simulink model "CoastdownCaCum1AQ_Ver2"  (R2024b)
settings: Solver=FixedStepAuto  StartTime=0  StopTime=14.2  FixedStep=0.2  RelTol=1e-3  AbsTol=1e-3  EnableMultiTasking=on
values from neighbouring files (symbols this model uses):
  a01 = 0.2657    [BCS_CoastdownCaCum1AQ_Ver2_lan2.mat]    (also in BCS_CoastdownCaCum2AQ_Ver2_lan2.mat)
  a02 = 0.0601    [BCS_CoastdownCaCum1AQ_Ver2_lan2.mat]    (also in BCS_CoastdownCaCum2AQ_Ver2_lan2.mat)
  a11 = 0.0614452785671    [BCS_CoastdownCaCum1AQ_Ver2_lan2.mat]    (also in BCS_CoastdownCaCum2AQ_Ver2_lan2.mat = 0.063131954008; CodeSosanhtonhaophatsinh_coastdown.m = alpha(1,1))
  a12 = 0.00726010495763    [BCS_CoastdownCaCum1AQ_Ver2_lan2.mat]    (also in BCS_CoastdownCaCum2AQ_Ver2_lan2.mat = 0.00749561097786; CodeSosanhtonhaophatsinh_coastdown.m = alpha(1,3))
  b01 = 6.7129    [BCS_CoastdownCaCum1AQ_Ver2_lan2.mat]    (also in BCS_CoastdownCaCum2AQ_Ver2_lan2.mat)
  b02 = 8.2494    [BCS_CoastdownCaCum1AQ_Ver2_lan2.mat]    (also in BCS_CoastdownCaCum2AQ_Ver2_lan2.mat)
  b11 = 1.46186355306    [BCS_CoastdownCaCum1AQ_Ver2_lan2.mat]    (also in BCS_CoastdownCaCum2AQ_Ver2_lan2.mat = 1.7584586215; CodeSosanhtonhaophatsinh_coastdown.m = alpha(1,2))
  b12 = 0.148893725861    [BCS_CoastdownCaCum1AQ_Ver2_lan2.mat]    (also in BCS_CoastdownCaCum2AQ_Ver2_lan2.mat = 0.267310835842; CodeSosanhtonhaophatsinh_coastdown.m = alpha(1,4))
  J_bx = 0.2412    [BCS_CoastdownCaCum1AQ_Ver2_lan2.mat]    (also in BCS_CoastdownCaCum2AQ_Ver2_lan2.mat)
  J_cl = 1.2576    [BCS_CoastdownCaCum1AQ_Ver2_lan2.mat]    (also in BCS_CoastdownCaCum2AQ_Ver2_lan2.mat)
  r_bx = 0.236102    [BCS_CoastdownCaCum1AQ_Ver2_lan2.mat]    (also in BCS_CoastdownCaCum2AQ_Ver2_lan2.mat = 0.235146)
  r_cl = 0.1    [BCS_CoastdownCaCum1AQ_Ver2_lan2.mat]    (also in BCS_CoastdownCaCum2AQ_Ver2_lan2.mat)
  Trr = 0.35615623487    [BCS_CoastdownCaCum1AQ_Ver2_lan2.mat]    (also in BCS_CoastdownCaCum2AQ_Ver2_lan2.mat = 0.370900243988; CodeSosanhtonhaophatsinh_coastdown.m = alpha(1,5))
  w_cl_initial = 55.8852681159    [BCS_CoastdownCaCum1AQ_Ver2_lan2.mat]    (also in BCS_CoastdownCaCum2AQ_Ver2_lan2.mat = 55.880555727; CodeSosanhtonhaophatsinh_coastdown.m = n_cl_tn(1,1)*2*pi()/60)
undefined symbols (not defined in the file or in its folder): rad, s
libraries: aerolibconvert2 x2, SignalEditorBlockLib x1
settings Model: Creator=Admin  LastModifiedBy=Legion
settings SolverCC: AutoScaleAbsTol=off  AlgebraicLoopSolver=TrustRegion  MaxZcPerStep=1
settings DataIOCC: LimitDataPoints=on  MaxDataPoints=10000
settings OptimizationCC: ReuseModelBlockBuffer=off  LifeSpan=inf
settings DebuggingCC: UnconnectedInputMsg=warning  UnconnectedOutputMsg=warning  UnconnectedLineMsg=warning  AllowSymbolicDim=off  SubsystemReferenceDiagnosticForUnitTest=warning  SFUnexpectedBacktrackingDiag=warning  SFNoUnconditionalDefaultTransitionDiag=warning  SFExecutionAtInitializationDiag=none  ArithmeticOperatorsInVariantConditions=warning
settings ModelReferenceCC: EnableRefExpFcnMdlSchedulingChecks=on
settings SFSimCC: SimUseLocalCustomCode=off  CustomCodeUndefinedFunction=UseInterfaceOnly
settings RTWCC: RTWUseLocalCustomCode=off  GPUComputeCapability=3.5  DLArmComputeVersion=19.05
settings CodeAppCC: StateflowObjectComments=on
settings GRTTargetCC: TargetLangStandard=C89/C90 (ANSI)
settings ConfigComp: CovMetricSettings=dw  CovSaveCumulativeToWorkspaceVar=on  CovSaveSingleToWorkspaceVar=on  CovExternalEMLEnable=off  CovSFcnEnable=off
settings SimscapeCC: SimscapeLogType=all  SimscapeLogSimulationStatistics=on  SimscapeLogDataHistory=10000

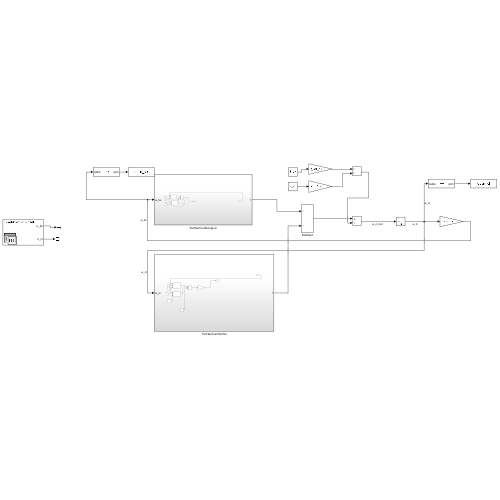
[thumbnail: Simulink's stored preview of the top-level diagram]
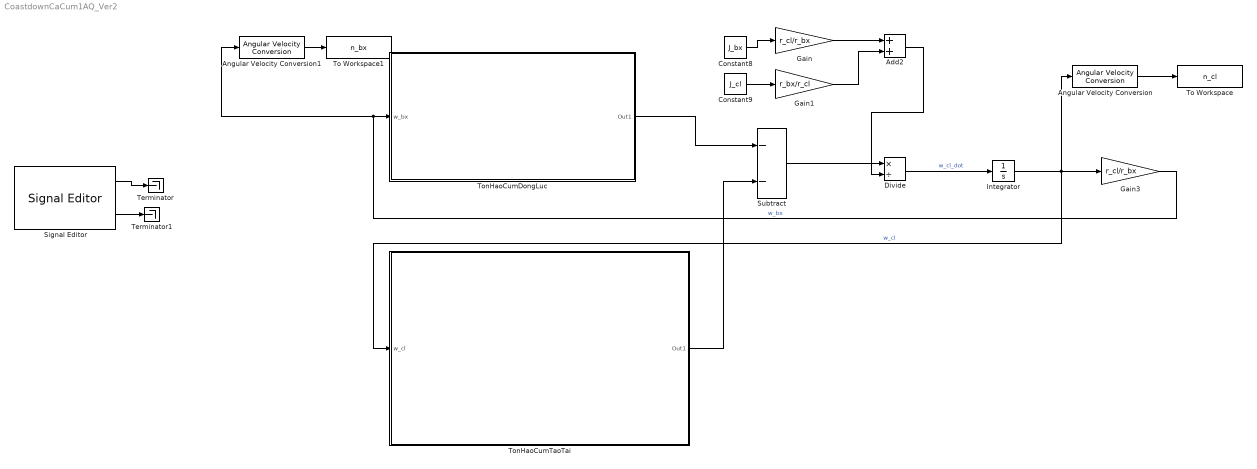
== system CoastdownCaCum1AQ_Ver2 ==
  Add2 : Sum
  Angular Velocity Conversion : aerolibconvert2/Angular Velocity Conversion  IU=rad/s  OU=rpm
  Angular Velocity Conversion1 : aerolibconvert2/Angular Velocity Conversion  IU=rad/s  OU=rpm
  Constant8 : Constant  Value=J_bx
  Constant9 : Constant  Value=J_cl  VectorParams1D=off
  Divide : Product  Inputs=*/
  Gain : Gain  Gain=r_cl/r_bx
  Gain1 : Gain  Gain=r_bx/r_cl
  Gain3 : Gain  Gain=r_cl/r_bx
  Integrator : Integrator  InitialCondition=w_cl_initial  LimitOutput=on  LowerSaturationLimit=0
  Signal Editor : SignalEditorBlockLib/Signal Editor  FileName=DataCoastdownCacum1AQchoSignalEditor.mat  ActiveScenario=CoastdownCaCum1AQ  ActiveSignal=n_bx  IsBus=off  OutputBusObjectStr=Bus: BusObject  SampleTime=0  ZeroCross=off  OutputAfterFinalValue=Setting to zero  Unit=inherit  PreserveSignalName=on  ApplySigPropsToAllScenarios=on  ApplySigPropsToAllSignals=off
  Subtract : Sum  Inputs=--
  Terminator : Terminator
  Terminator1 : Terminator
  To Workspace : ToWorkspace  VariableName=n_cl  SaveFormat=Timeseries  SampleTime=-1
  To Workspace1 : ToWorkspace  VariableName=n_bx  SaveFormat=Timeseries  SampleTime=-1
  TonHaoCumDongLuc : Subsystem
  TonHaoCumTaoTai : Subsystem
  wires:
  Subtract/1 -> Divide/1
  Signal Editor/1 -> Terminator/1
  Signal Editor/2 -> Terminator1/1
  Constant8/1 -> Gain/1
  Constant9/1 -> Gain1/1
  Gain/1 -> Add2/1
  Gain1/1 -> Add2/2
  Add2/1 -> Divide/2
  Divide/1 -> Integrator/1  "w_cl_dot"
  Integrator/1 -> TonHaoCumTaoTai/1(w_cl), Angular Velocity Conversion/1, Gain3/1  "w_cl"
  Angular Velocity Conversion/1 -> To Workspace/1
  TonHaoCumTaoTai/1(Out1) -> Subtract/2
  Gain3/1 -> TonHaoCumDongLuc/1(w_bx), Angular Velocity Conversion1/1  "w_bx"
  TonHaoCumDongLuc/1(Out1) -> Subtract/1
  Angular Velocity Conversion1/1 -> To Workspace1/1

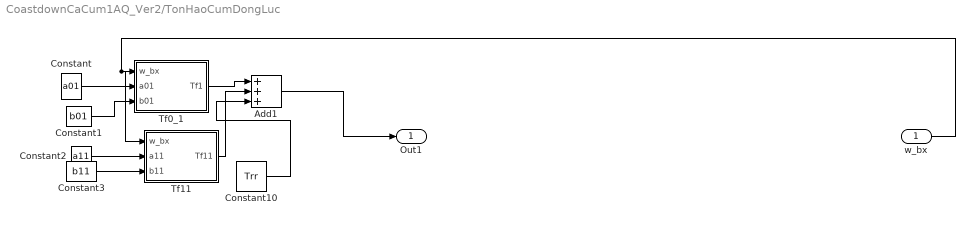
== system CoastdownCaCum1AQ_Ver2/TonHaoCumDongLuc ==
  w_bx : Inport
  Add1 : Sum  Inputs=+++
  Constant : Constant  Value=a01
  Constant1 : Constant  Value=b01
  Constant10 : Constant  Value=Trr
  Constant2 : Constant  Value=a11
  Constant3 : Constant  Value=b11
  Tf0_1 : MATLAB Function  TreatAsAtomicUnit=on
  Tf11 : MATLAB Function  TreatAsAtomicUnit=on
  Out1 : Outport
  wires:
  w_bx/1 -> Tf11/1(w_bx), Tf0_1/1(w_bx)
  Constant/1 -> Tf0_1/2(a01)
  Constant1/1 -> Tf0_1/3(b01)
  Constant3/1 -> Tf11/3(b11)
  Constant2/1 -> Tf11/2(a11)
  Tf0_1/1(Tf1) -> Add1/1
  Tf11/1(Tf11) -> Add1/2
  Constant10/1 -> Add1/3
  Add1/1 -> Out1/1

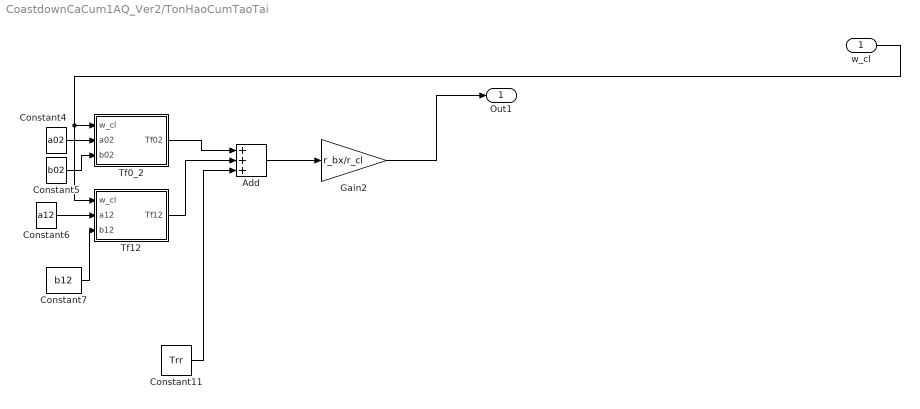
== system CoastdownCaCum1AQ_Ver2/TonHaoCumTaoTai ==
  w_cl : Inport
  Add : Sum  Inputs=+++
  Constant11 : Constant  Value=Trr
  Constant4 : Constant  Value=a02
  Constant5 : Constant  Value=b02
  Constant6 : Constant  Value=a12
  Constant7 : Constant  Value=b12
  Gain2 : Gain  Gain=r_bx/r_cl
  Tf0_2 : MATLAB Function  TreatAsAtomicUnit=on
  Tf12 : MATLAB Function  TreatAsAtomicUnit=on
  Out1 : Outport
  wires:
  Tf12/1(Tf12) -> Add/2
  Constant5/1 -> Tf0_2/3(b02)
  Constant6/1 -> Tf12/2(a12)
  Constant4/1 -> Tf0_2/2(a02)
  Tf0_2/1(Tf02) -> Add/1
  Constant7/1 -> Tf12/3(b12)
  Constant11/1 -> Add/3
  Add/1 -> Gain2/1
  w_cl/1 -> Tf12/1(w_cl), Tf0_2/1(w_cl)
  Gain2/1 -> Out1/1

== matlab function CoastdownCaCum1AQ_Ver2/TonHaoCumDongLuc/Tf0_1 ==
  data: w_bx input; Tf1 output; a01 input; b01 input
function Tf1 = fcn(w_bx,a01,b01)

Tf1 = 0.0362*(a01*w_bx+b01)*15;

== matlab function CoastdownCaCum1AQ_Ver2/TonHaoCumDongLuc/Tf11 ==
  data: w_bx input; Tf11 output; a11 input; b11 input
function Tf11 = fcn(w_bx,a11,b11)

Tf11 = a11*w_bx+b11;

== matlab function CoastdownCaCum1AQ_Ver2/TonHaoCumTaoTai/Tf12 ==
  data: w_cl input; Tf12 output; a12 input; b12 input
function Tf12 = fcn(w_cl,a12,b12)

Tf12 = a12*w_cl+b12;

== matlab function CoastdownCaCum1AQ_Ver2/TonHaoCumTaoTai/Tf0_2 ==
  data: w_cl input; Tf02 output; a02 input; b02 input
function Tf02 = fcn(w_cl,a02,b02)

Tf02 = 0.0362*(a02*w_cl+b02)*2;
